simulink model "FSFB_Int_Controller"  (R2022a)
settings: Solver=VariableStepAuto  StartTime=0.0  StopTime=10.0  RelTol=1e-3
undefined symbols (not defined in the file): K1, K2
settings Model: Creator=domin  LastModifiedBy=domin

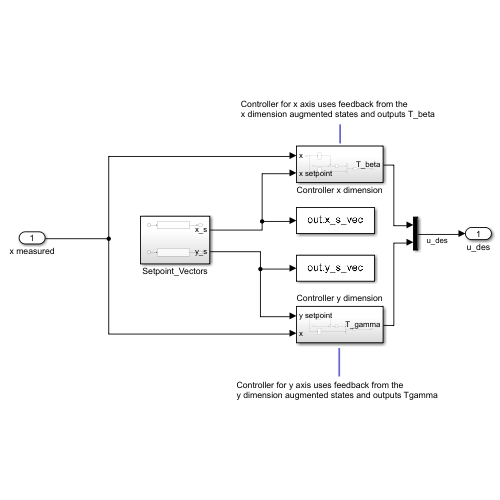
[thumbnail: Simulink's stored preview of the top-level diagram]
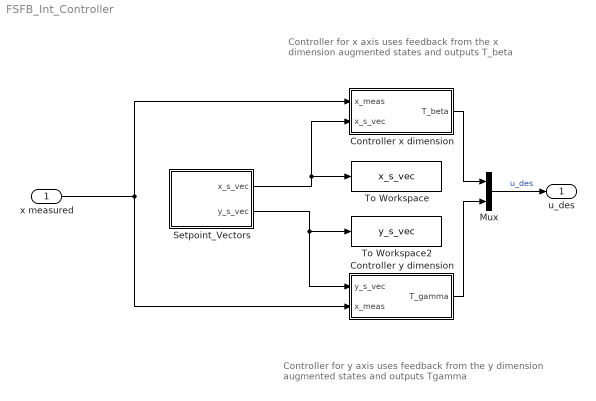
== system FSFB_Int_Controller ==
  note: Controller for y axis uses feedback from the
      | y dimension augmented states and outputs Tgamma
  note: Controller for x axis uses feedback from the
      | x dimension augmented states and outputs T_beta
  x measured : Inport
  Controller x dimension : Subsystem
  Controller y dimension : Subsystem
  Mux : Mux  Inputs=2
  Setpoint_Vectors : Subsystem
  To Workspace : ToWorkspace  VariableName=x_s_vec  SampleTime=-1
  To Workspace2 : ToWorkspace  VariableName=y_s_vec  SampleTime=-1
  u_des : Outport
  wires:
  Mux/1 -> u_des/1  "u_des"
  Setpoint_Vectors/1(x_s_vec) -> Controller x dimension/2(x_s_vec), To Workspace/1
  Controller y dimension/1(T_gamma) -> Mux/2
  Controller x dimension/1(T_beta) -> Mux/1
  Setpoint_Vectors/2(y_s_vec) -> Controller y dimension/1(y_s_vec), To Workspace2/1
  x measured/1 -> Controller x dimension/1(x_meas), Controller y dimension/2(x_meas)

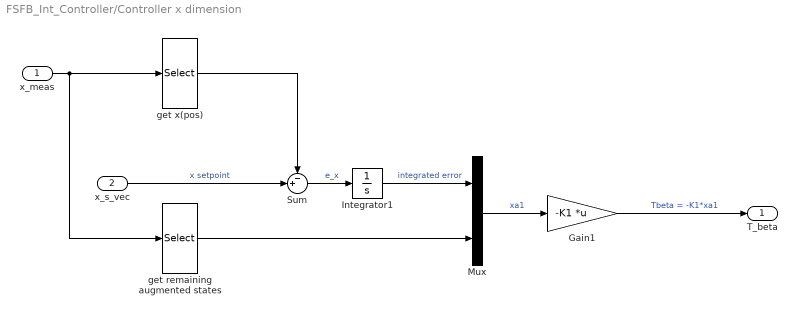
== system FSFB_Int_Controller/Controller x dimension ==
  x_meas : Inport
  x_s_vec : Inport  Port=2
  Gain1 : Gain  Gain=-K1  Multiplication=Matrix(K*u)
  Integrator1 : Integrator
  Mux : Mux  Inputs=2
  Sum : Sum  Inputs=-+|
  get remaining augmented states : Selector  InputPortWidth=8  IndexOptions=Index vector (dialog)  Indices=[1,2,3,4]  OutputSizes=1
  get x(pos) : Selector  InputPortWidth=8  IndexOptions=Index vector (dialog)  Indices=[1]  OutputSizes=1
  T_beta : Outport
  wires:
  get remaining augmented states/1 -> Mux/2
  Gain1/1 -> T_beta/1  "Tbeta = -K1*xa1"
  get x(pos)/1 -> Sum/1
  Mux/1 -> Gain1/1  "xa1"
  Sum/1 -> Integrator1/1  "e_x"
  Integrator1/1 -> Mux/1  "integrated error"
  x_s_vec/1 -> Sum/2  "x setpoint"
  x_meas/1 -> get remaining augmented states/1, get x(pos)/1

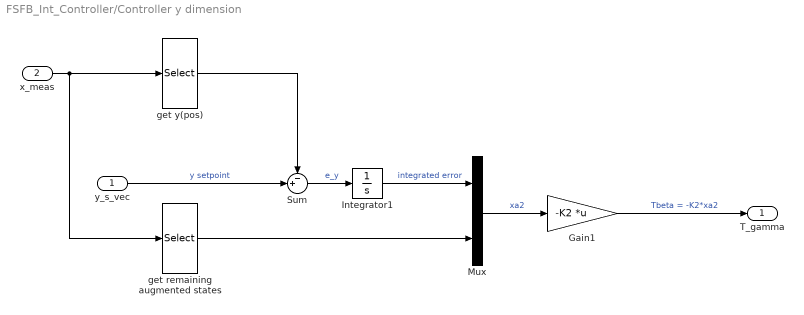
== system FSFB_Int_Controller/Controller y dimension ==
  y_s_vec : Inport
  x_meas : Inport  Port=2
  Gain1 : Gain  Gain=-K2  Multiplication=Matrix(K*u)
  Integrator1 : Integrator
  Mux : Mux  Inputs=2
  Sum : Sum  Inputs=-+|
  get remaining augmented states : Selector  InputPortWidth=8  IndexOptions=Index vector (dialog)  Indices=[5,6,7,8]  OutputSizes=1
  get y(pos) : Selector  InputPortWidth=8  IndexOptions=Index vector (dialog)  Indices=[2]  OutputSizes=1
  T_gamma : Outport
  wires:
  x_meas/1 -> get y(pos)/1, get remaining augmented states/1
  y_s_vec/1 -> Sum/2  "y setpoint"
  Integrator1/1 -> Mux/1  "integrated error"
  Sum/1 -> Integrator1/1  "e_y"
  Mux/1 -> Gain1/1  "xa2"
  get y(pos)/1 -> Sum/1
  Gain1/1 -> T_gamma/1  "Tbeta = -K2*xa2"
  get remaining augmented states/1 -> Mux/2

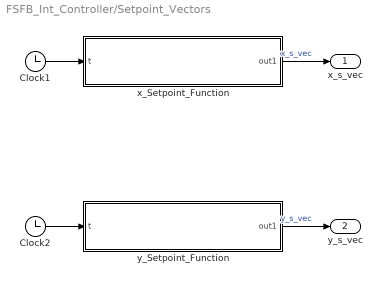
== system FSFB_Int_Controller/Setpoint_Vectors ==
  Clock1 : Clock
  Clock2 : Clock
  x_Setpoint_Function : MATLAB Function  TreatAsAtomicUnit=on
  y_Setpoint_Function : MATLAB Function  TreatAsAtomicUnit=on
  x_s_vec : Outport
  y_s_vec : Outport  Port=2
  wires:
  y_Setpoint_Function/1(out1) -> y_s_vec/1  "y_s_vec"
  Clock2/1 -> y_Setpoint_Function/1(t)
  Clock1/1 -> x_Setpoint_Function/1(t)
  x_Setpoint_Function/1(out1) -> x_s_vec/1  "x_s_vec"

== matlab function FSFB_Int_Controller/Setpoint_Vectors/y_Setpoint_Function ==
  data: t input; out1 output
function out1 = y_s_vec(t)
%#codegen

%    This function was generated by the Symbolic Math Toolbox version 9.1.
%    26-Nov-2022 21:59:45

t2 = t.*pi;
out1 = sin(t2./3.0).*(-3.0./4.0e+1)+sin(t2).*(3.0./4.0e+1);

== matlab function FSFB_Int_Controller/Setpoint_Vectors/x_Setpoint_Function ==
  data: t input; out1 output
function out1 = x_s_vec(t)
%#codegen

%    This function was generated by the Symbolic Math Toolbox version 9.1.
%    26-Nov-2022 21:59:45

t2 = t.*pi;
out1 = cos(t2./3.0).*(3.0./4.0e+1)+cos(t2).*(3.0./4.0e+1);
